simulink model "Hinf_1DOF_simulation"  (R2023a)
settings: Solver=VariableStepAuto  StartTime=0.0  StopTime=50  RelTol=1e-3
InitFcn:
  | Hinf_1DOF
values from neighbouring files (symbols this model uses):
  fa_w = 0    [Hinf_1DOF.m]    (also in Hinf_2DOFinit.m; Hinf_U_init.m; Hinf_WU_init.m; Hinf_init.m)
  fm_w = s_param.g*s_param.m    [Hinf_1DOF.m]    (also in Hinf_2DOFinit.m; Hinf_U_init.m; Hinf_WU_init.m; Hinf_init.m)
  K = tf(ss(K.A,K.B,K.C,K.D))    [Hinf_U_init.m]    (also in Hinf_WU_init.m; Hinf_init.m)
  Plant = ss(G)    [Hinf_1DOF.m]
  theta_w = 0    [Hinf_1DOF.m]    (also in Hinf_2DOFinit.m; Hinf_U_init.m; Hinf_WU_init.m; Hinf_init.m)
  x_0_real = [z_0_real; theta_0_real; dz_0_real; dtheta_0_real]    [Hinf_1DOF.m]    (also in Hinf_2DOFinit.m; Hinf_U_init.m; Hinf_WU_init.m; Hinf_init.m)
  z_w = 200    [Hinf_1DOF.m]    (also in Hinf_2DOFinit.m = 400; Hinf_U_init.m = 400; Hinf_WU_init.m = 400; Hinf_init.m = 400)
settings Model: Creator=franc  LastModifiedBy=rvitt

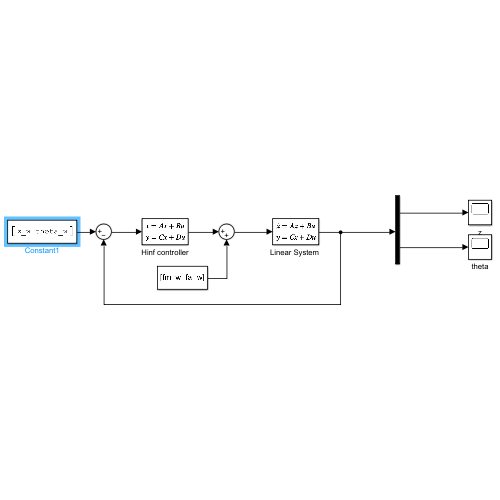
[thumbnail: Simulink's stored preview of the top-level diagram]
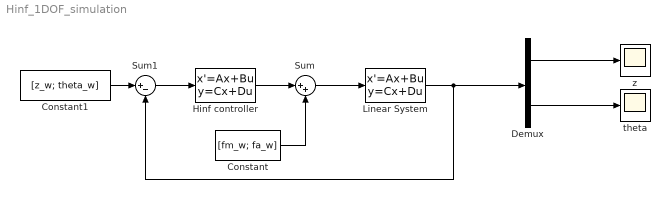
== system Hinf_1DOF_simulation ==
  Constant : Constant  Value=[fm_w; fa_w]
  Constant1 : Constant  Value=[z_w; theta_w]
  Demux : Demux  Outputs=2
  Hinf controller : StateSpace  A=K.A  B=K.B  C=K.C  D=K.D  InitialCondition=zeros(12,1)  ParameterTunability=Optimized
  "Linear System " : StateSpace  A=Plant.A  B=Plant.B  C=Plant.C  D=Plant.D  InitialCondition=[x_0_real; 0; 0; 0; 0; 0; 0;]  ParameterTunability=Optimized
  Sum : Sum  Inputs=|++
  Sum1 : Sum  Inputs=|+-
  theta : Scope
  z : Scope
  wires:
  Hinf controller/1 -> Sum/1
  "Linear System "/1 -> Sum1/2, Demux/1
  Demux/1 -> z/1
  Sum/1 -> "Linear System "/1
  Constant/1 -> Sum/2
  Demux/2 -> theta/1
  Constant1/1 -> Sum1/1
  Sum1/1 -> Hinf controller/1
